simulink model "array_calculations"  (R2021a)
settings: Solver=FixedStepDiscrete  StartTime=0.0  StopTime=10.0  RelTol=1e-3
settings Model: Creator=Dell  LastModifiedBy=Dell
settings OptimizationCC: DefaultParameterBehavior=Inlined  EnhancedBackFolding=on  PassReuseOutputArgsAs=Individual arguments  ZeroExternalMemoryAtStartup=off  ZeroInternalMemoryAtStartup=off  OptimizeBlockOrder=speed  DifferentSizesBufferReuse=on  OptimizationCustomize=off  EfficientTunableParamExpr=on
settings DebuggingCC: ParameterTunabilityLossMsg=error
settings SFSimCC: MATLABDynamicMemAlloc=off
settings RTWCC: SystemTargetFile=ert.tlc  GenCodeOnly=on  TemplateMakefile=ert_default_tmf  GenerateReport=on  IncludeHyperlinkInReport=on  LaunchReport=on  GenerateTraceInfo=on
settings CodeAppCC: ForceParamTrailComments=on  IgnoreCustomStorageClasses=off  OperatorAnnotations=on  SimulinkDataObjDesc=on  SFDataObjDesc=on  InsertBlockDesc=on
settings ERTTargetCC: TargetLangStandard=C99 (ISO)  GenerateSampleERTMain=on  InlinedParameterPlacement=NonHierarchical  ERTCustomFileTemplate=example_file_process.tlc

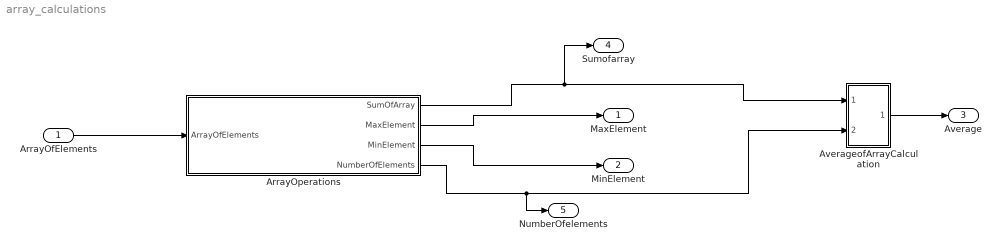
== system array_calculations ==
  ArrayOfElements : Inport
  ArrayOperations : Subsystem
  AverageofArrayCalculation : Subsystem
  MaxElement : Outport
  MinElement : Outport  Port=2
  Average : Outport  Port=3
  Sumofarray : Outport  Port=4
  NumberOfelements : Outport  Port=5
  wires:
  ArrayOfElements/1 -> ArrayOperations/1(ArrayOfElements)
  ArrayOperations/2(MaxElement) -> MaxElement/1
  ArrayOperations/3(MinElement) -> MinElement/1
  ArrayOperations/1(SumOfArray) -> Sumofarray/1, AverageofArrayCalculation/1(In1)
  ArrayOperations/4(NumberOfElements) -> NumberOfelements/1, AverageofArrayCalculation/2(In2)
  AverageofArrayCalculation/1(Out1) -> Average/1

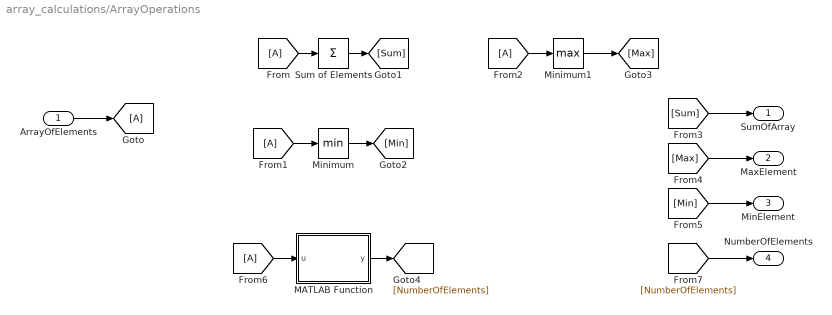
== system array_calculations/ArrayOperations ==
  ArrayOfElements : Inport  PortDimensions=[10]
  MATLAB Function : MATLAB Function  TreatAsAtomicUnit=on
  Minimum : MinMax
  Minimum1 : MinMax  Function=max
  Sum of Elements : Sum  Inputs=+
  SumOfArray : Outport
  MaxElement : Outport  Port=2
  MinElement : Outport  Port=3
  NumberOfElements : Outport  Port=4
  wires:
  [Max] -> MaxElement/1
  Minimum/1 -> [Min]
  [A] -> MATLAB Function/1(u)
  [A] -> Minimum/1
  [A] -> Sum of Elements/1
  [Sum] -> SumOfArray/1
  [NumberOfElements] -> NumberOfElements/1
  MATLAB Function/1(y) -> [NumberOfElements]
  ArrayOfElements/1 -> [A]
  Sum of Elements/1 -> [Sum]
  [Min] -> MinElement/1
  Minimum1/1 -> [Max]
  [A] -> Minimum1/1

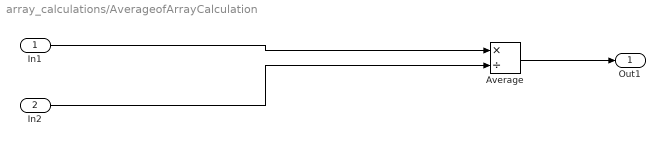
== system array_calculations/AverageofArrayCalculation ==
  In1 : Inport
  In2 : Inport  Port=2
  Average : Product  Inputs=*/
  Out1 : Outport
  wires:
  In2/1 -> Average/2
  Average/1 -> Out1/1
  In1/1 -> Average/1

== matlab function array_calculations/ArrayOperations/MATLAB Function ==
  data: u input; y output
function y = fcn(u)
% Use numel function to count the number of elements
    y = numel(u);
end
